simulink model "PI_controller"  (R2020a)
settings: Solver=VariableStepAuto  StartTime=0.0  StopTime=10.0  RelTol=1e-3
settings Model: Creator=Administrator  LastModifiedBy=Administrator

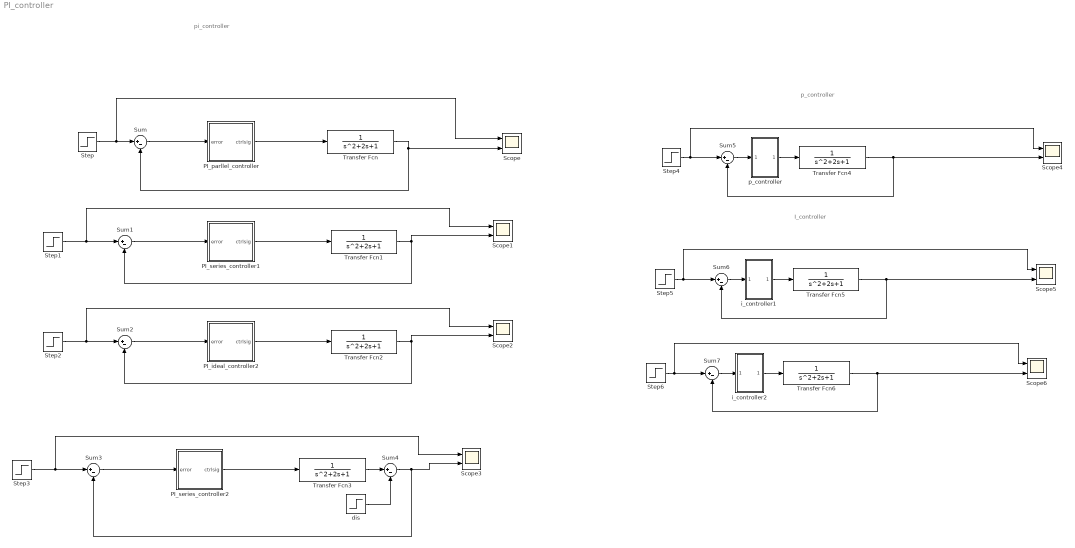
== system PI_controller ==
  note: p_controller
  note: pi_controller
  note: I_controller
  PI_ideal_controller2 : Subsystem
  PI_parllel_controller : Subsystem
  PI_series_controller1 : Subsystem
  PI_series_controller2 : Subsystem
  Scope{,1..6} (7 alike) : Scope  NumInputPorts=2
  Step{,1..6} (7 alike) : Step  SampleTime=0
  Sum{,1..7} (8 alike) : Sum  Inputs=|+-
  Transfer Fcn{,1..6} (7 alike) : TransferFcn
  dis : Step  Time=4  SampleTime=0
  i_controller1 : Subsystem
  i_controller2 : Subsystem
  p_controller : Subsystem
  wires:
  PI_parllel_controller/1(ctrlsig) -> Transfer Fcn/1
  Transfer Fcn/1 -> Scope/2, Sum/2
  Sum/1 -> PI_parllel_controller/1(error)
  Step/1 -> Scope/1, Sum/1
  PI_series_controller1/1(ctrlsig) -> Transfer Fcn1/1
  Step1/1 -> Scope1/1, Sum1/1
  Sum1/1 -> PI_series_controller1/1(error)
  Transfer Fcn1/1 -> Scope1/2, Sum1/2
  Transfer Fcn2/1 -> Sum2/2, Scope2/2
  Sum2/1 -> PI_ideal_controller2/1(error)
  Step2/1 -> Sum2/1, Scope2/1
  PI_ideal_controller2/1(ctrlsig) -> Transfer Fcn2/1
  Sum3/1 -> PI_series_controller2/1(error)
  Step3/1 -> Sum3/1, Scope3/1
  PI_series_controller2/1(ctrlsig) -> Transfer Fcn3/1
  Transfer Fcn3/1 -> Sum4/1
  dis/1 -> Sum4/2
  Sum4/1 -> Scope3/2, Sum3/2
  Step4/1 -> Sum5/1, Scope4/1
  Transfer Fcn4/1 -> Sum5/2, Scope4/2
  Sum5/1 -> p_controller/1(In1)
  p_controller/1(Out1) -> Transfer Fcn4/1
  i_controller1/1(Out1) -> Transfer Fcn5/1
  Sum6/1 -> i_controller1/1(In1)
  Transfer Fcn5/1 -> Scope5/2, Sum6/2
  Step5/1 -> Scope5/1, Sum6/1
  Step6/1 -> Sum7/1, Scope6/1
  Transfer Fcn6/1 -> Sum7/2, Scope6/2
  Sum7/1 -> i_controller2/1(In1)
  i_controller2/1(Out1) -> Transfer Fcn6/1

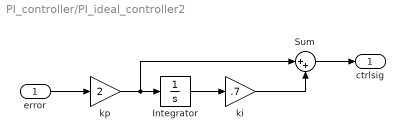
== system PI_controller/PI_ideal_controller2 ==
  error : Inport
  Integrator : Integrator
  Sum : Sum  Inputs=|++
  ki : Gain  Gain=.7
  kp : Gain  Gain=2
  ctrlsig : Outport
  wires:
  Integrator/1 -> ki/1
  ki/1 -> Sum/2
  error/1 -> kp/1
  Sum/1 -> ctrlsig/1
  kp/1 -> Integrator/1, Sum/1

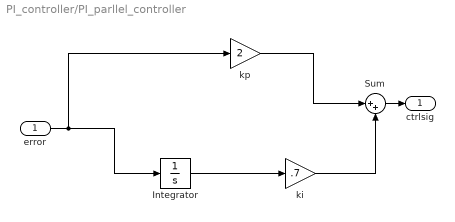
== system PI_controller/PI_parllel_controller ==
  error : Inport
  Integrator : Integrator
  Sum : Sum  Inputs=|++
  ki : Gain  Gain=.7
  kp : Gain  Gain=2
  ctrlsig : Outport
  wires:
  kp/1 -> Sum/1
  ki/1 -> Sum/2
  error/1 -> kp/1, Integrator/1
  Integrator/1 -> ki/1
  Sum/1 -> ctrlsig/1

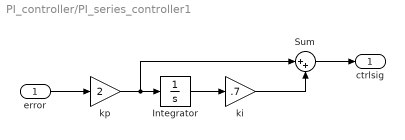
== system PI_controller/PI_series_controller1 ==
  error : Inport
  Integrator : Integrator
  Sum : Sum  Inputs=|++
  ki : Gain  Gain=.7
  kp : Gain  Gain=2
  ctrlsig : Outport
  wires:
  kp/1 -> Sum/1, Integrator/1
  Sum/1 -> ctrlsig/1
  error/1 -> kp/1
  ki/1 -> Sum/2
  Integrator/1 -> ki/1

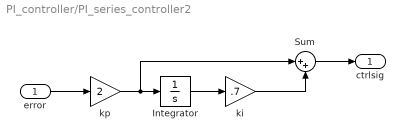
== system PI_controller/PI_series_controller2 ==
  error : Inport
  Integrator : Integrator
  Sum : Sum  Inputs=|++
  ki : Gain  Gain=.7
  kp : Gain  Gain=2
  ctrlsig : Outport
  wires:
  Integrator/1 -> ki/1
  ki/1 -> Sum/2
  error/1 -> kp/1
  Sum/1 -> ctrlsig/1
  kp/1 -> Integrator/1, Sum/1

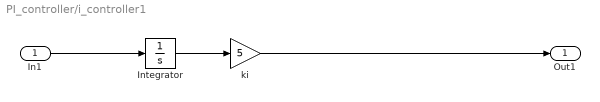
== system PI_controller/i_controller1 ==
  In1 : Inport
  Integrator : Integrator
  ki : Gain  Gain=5
  Out1 : Outport
  wires:
  ki/1 -> Out1/1
  In1/1 -> Integrator/1
  Integrator/1 -> ki/1

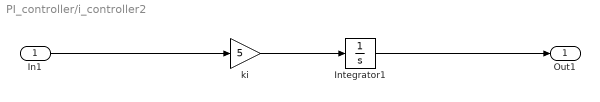
== system PI_controller/i_controller2 ==
  In1 : Inport
  Integrator1 : Integrator
  ki : Gain  Gain=5
  Out1 : Outport
  wires:
  In1/1 -> ki/1
  ki/1 -> Integrator1/1
  Integrator1/1 -> Out1/1

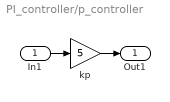
== system PI_controller/p_controller ==
  In1 : Inport
  kp : Gain  Gain=5
  Out1 : Outport
  wires:
  In1/1 -> kp/1
  kp/1 -> Out1/1
